simulink model "model_king"  (R2017a)
settings: Solver=VariableStepAuto  StartTime=0.0  StopTime=10.0  RelTol=1e-3
undefined symbols (not defined in the file): g, m, wind
settings Model: Creator=My  LastModifiedBy=My

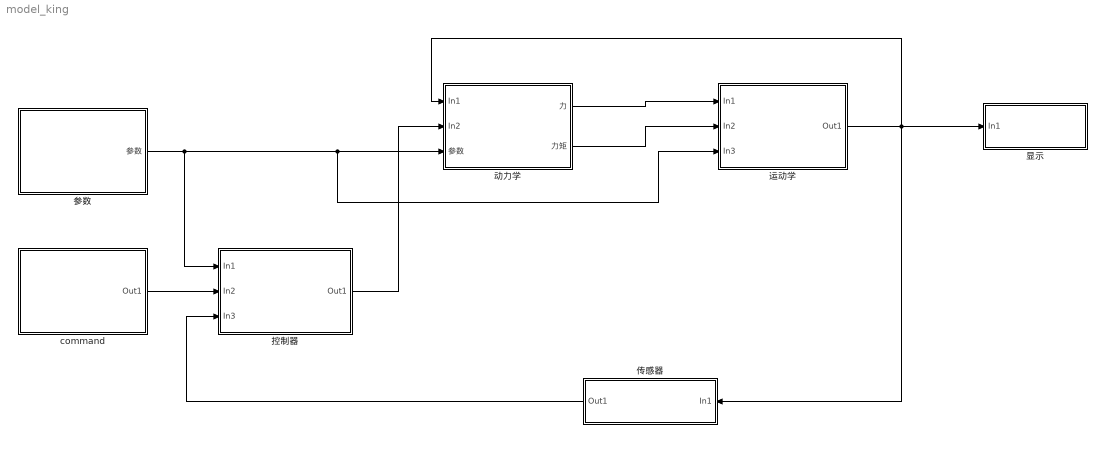
== system model_king ==
  "command " : Subsystem
  传感器 : Subsystem
  动力学 : Subsystem
  参数 : Subsystem
  控制器 : Subsystem
  显示 : Subsystem
  运动学 : Subsystem
  wires:
  运动学/1(Out1) -> 显示/1(In1), 传感器/1(In1), 动力学/1(In1)
  参数/1(参数) -> 控制器/1(In1), 运动学/3(In3), 动力学/3(参数)
  控制器/1(Out1) -> 动力学/2(In2)
  "command "/1(Out1) -> 控制器/2(In2)
  传感器/1(Out1) -> 控制器/3(In3)
  动力学/1(力) -> 运动学/1(In1)
  动力学/2(力矩) -> 运动学/2(In2)

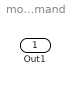
== system model_king/command  ==
  Out1 : Outport

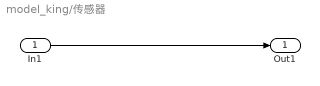
== system model_king/传感器 ==
  In1 : Inport
  Out1 : Outport
  wires:
  In1/1 -> Out1/1

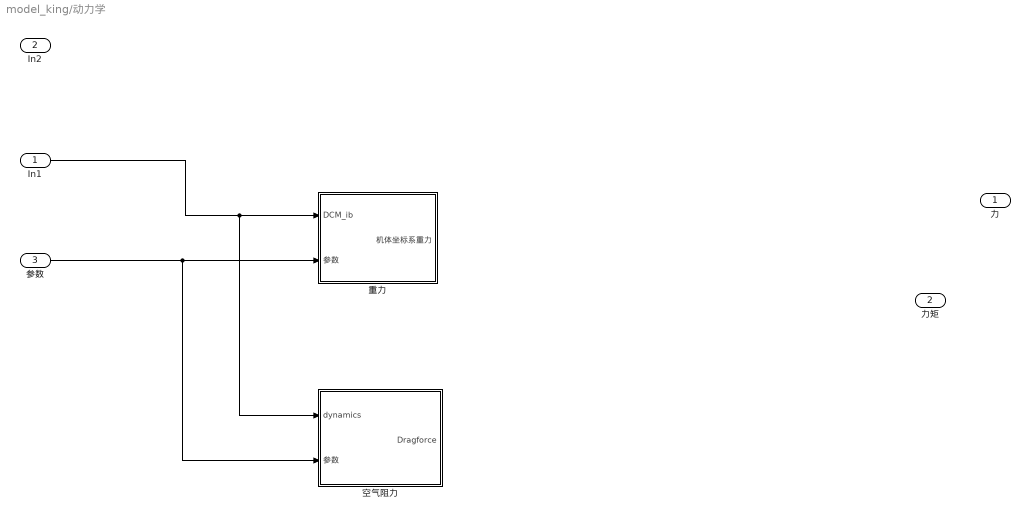
== system model_king/动力学 ==
  In1 : Inport
  In2 : Inport  Port=2
  参数 : Inport  Port=3
  空气阻力 : Subsystem
  重力 : Subsystem
  力 : Outport
  力矩 : Outport  Port=2
  wires:
  参数/1 -> 空气阻力/2(参数), 重力/2(参数)
  In1/1 -> 空气阻力/1(dynamics), 重力/1(DCM_ib)

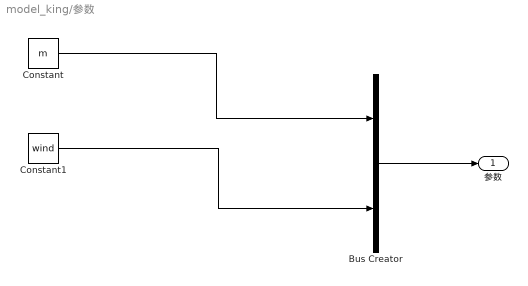
== system model_king/参数 ==
  Bus Creator : BusCreator  Inputs='m','wind_i'
  Constant : Constant  Value=m
  Constant1 : Constant  Value=wind
  参数 : Outport
  wires:
  Constant/1 -> Bus Creator/1
  Bus Creator/1 -> 参数/1
  Constant1/1 -> Bus Creator/2

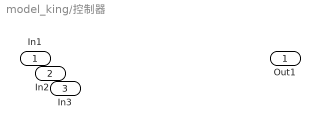
== system model_king/控制器 ==
  In1 : Inport
  In2 : Inport  Port=2
  In3 : Inport  Port=3
  Out1 : Outport

== system model_king/显示 ==
  In1 : Inport

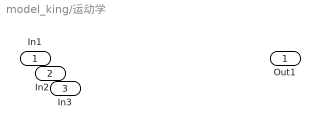
== system model_king/运动学 ==
  In1 : Inport
  In2 : Inport  Port=2
  In3 : Inport  Port=3
  Out1 : Outport

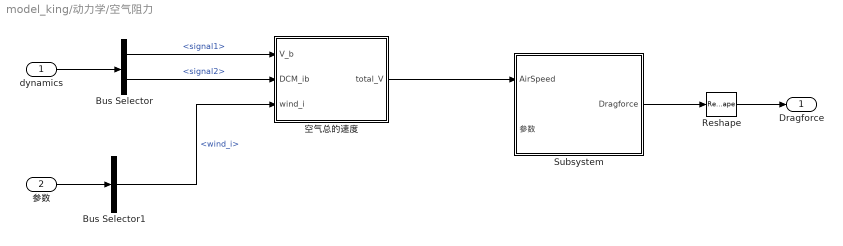
== system model_king/动力学/空气阻力 ==
  dynamics : Inport
  参数 : Inport  Port=2
  Bus Selector : BusSelector  OutputSignals=signal1,signal2
  Bus Selector1 : BusSelector  OutputSignals=wind_i
  Reshape : Reshape  OutputDimensionality=Column vector (2-D)
  Subsystem : Subsystem
  空气总的速度 : Subsystem
  Dragforce : Outport
  wires:
  dynamics/1 -> Bus Selector/1
  Bus Selector/1 -> 空气总的速度/1(V_b)  "<signal1>"
  Bus Selector/2 -> 空气总的速度/2(DCM_ib)  "<signal2>"
  参数/1 -> Bus Selector1/1
  Bus Selector1/1 -> 空气总的速度/3(wind_i)  "<wind_i>"
  空气总的速度/1(total_V) -> Subsystem/1(AirSpeed)
  Reshape/1 -> Dragforce/1
  Subsystem/1(Dragforce) -> Reshape/1

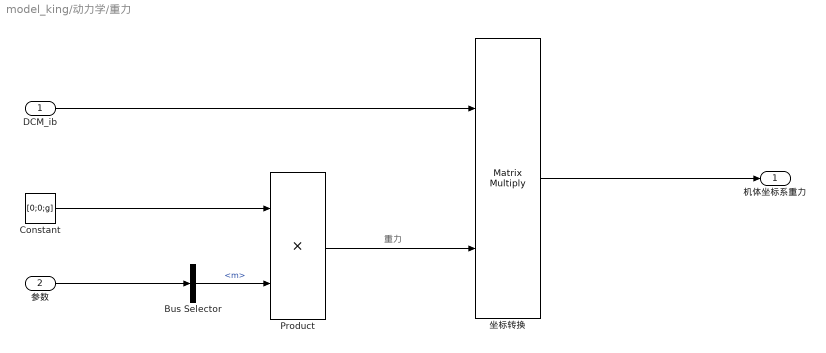
== system model_king/动力学/重力 ==
  note: 重力
  DCM_ib : Inport
  参数 : Inport  Port=2
  Bus Selector : BusSelector  OutputSignals=m
  Constant : Constant  Value=[0;0;g]
  Product : Product
  坐标转换 : Product  Multiplication=Matrix(*)
  机体坐标系重力 : Outport
  wires:
  参数/1 -> Bus Selector/1
  Constant/1 -> Product/1
  Bus Selector/1 -> Product/2  "<m>"
  Product/1 -> 坐标转换/2
  DCM_ib/1 -> 坐标转换/1
  坐标转换/1 -> 机体坐标系重力/1

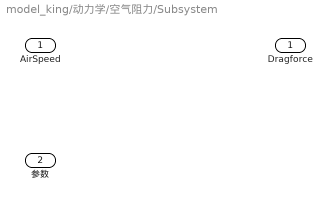
== system model_king/动力学/空气阻力/Subsystem ==
  AirSpeed : Inport
  参数 : Inport  Port=2
  Dragforce : Outport

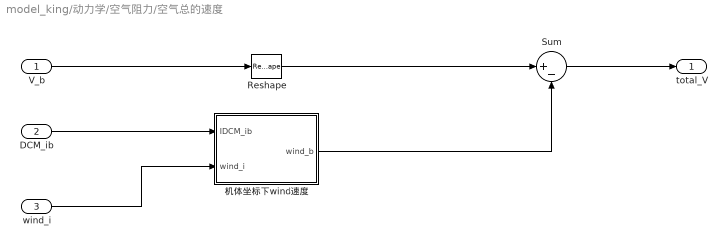
== system model_king/动力学/空气阻力/空气总的速度 ==
  V_b : Inport
  DCM_ib : Inport  Port=2
  wind_i : Inport  Port=3
  Reshape : Reshape  OutputDimensionality=Column vector (2-D)
  Sum : Sum  Inputs=|+-
  机体坐标下wind速度 : Subsystem
  total_V : Outport
  wires:
  V_b/1 -> Reshape/1
  DCM_ib/1 -> 机体坐标下wind速度/1(IDCM_ib)
  wind_i/1 -> 机体坐标下wind速度/2(wind_i)
  Reshape/1 -> Sum/1
  机体坐标下wind速度/1(wind_b) -> Sum/2
  Sum/1 -> total_V/1

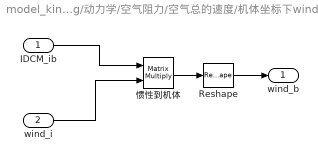
== system model_king/动力学/空气阻力/空气总的速度/机体坐标下wind速度 ==
  IDCM_ib : Inport
  wind_i : Inport  Port=2
  Reshape : Reshape  OutputDimensionality=Column vector (2-D)
  惯性到机体 : Product  Multiplication=Matrix(*)
  wind_b : Outport
  wires:
  IDCM_ib/1 -> 惯性到机体/1
  wind_i/1 -> 惯性到机体/2
  惯性到机体/1 -> Reshape/1
  Reshape/1 -> wind_b/1
